simulink model "ADEV_Sim"  (R2023b)
settings: Solver=VariableStepAuto  StartTime=0.0  StopTime=50000  RelTol=1e-3
libraries: simulink x1
settings Model: SimulationMode=accelerator  Creator=ijifl  LastModifiedBy=ijifl

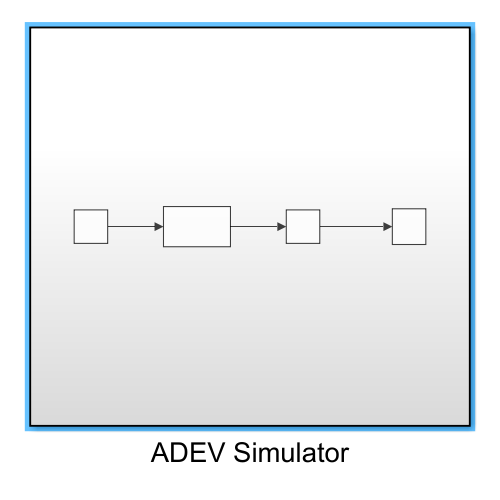
[thumbnail: Simulink's stored preview of the top-level diagram]
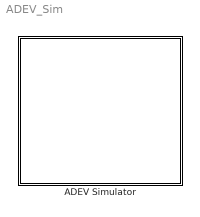
== system ADEV_Sim ==
  ADEV Simulator : Subsystem

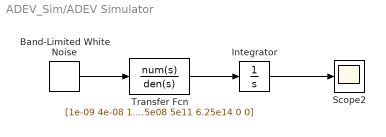
== system ADEV_Sim/ADEV Simulator ==
  Band-Limited White Noise : simulink/Sources/Band-Limited White Noise  Cov=[1]  Ts=0.1  seed=[23341]
  Integrator : Integrator
  Scope2 : Scope
  Transfer Fcn : TransferFcn  Numerator=[1e-09 4e-08 1.2e-11 1e-15 4e-20]  Denominator=[1 20000 1.5e08 5e11 6.25e14 0 0]
  wires:
  Transfer Fcn/1 -> Integrator/1
  Integrator/1 -> Scope2/1
  Band-Limited White Noise/1 -> Transfer Fcn/1
